simulink model "PowerCircuitPlant"  (R2020a)
settings: Solver=VariableStepAuto  StartTime=0.0  StopTime=10.0  RelTol=1e-3
libraries: fl_lib x5, nesl_utility x4, ee_lib x2
settings Model: DataDictionary=PCS_Simulation_EnviromentDD.sldd  Creator=ykamatan  LastModifiedBy=ykamatan

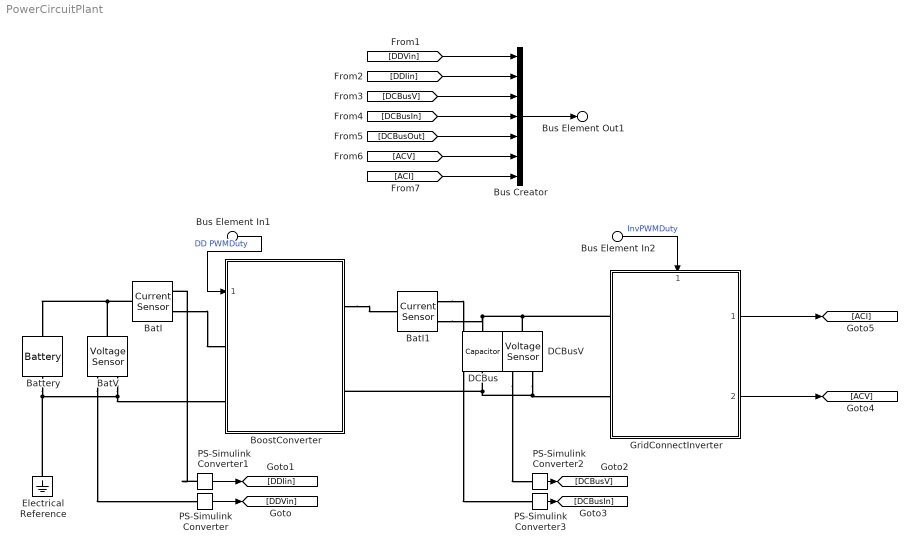
== system PowerCircuitPlant ==
  Bus Element In1 : Inport  PortName=DD PWMDuty
  Bus Element In2 : Inport  Port=2  PortName=InvPWMDuty
  BatI : fl_lib/Electrical/Electrical Sensors/Current Sensor
  BatI1 : fl_lib/Electrical/Electrical Sensors/Current Sensor
  BatV : fl_lib/Electrical/Electrical Sensors/Voltage Sensor
  Battery : ee_lib/Sources/Battery  Vnom=12 V  R1=2 Ohm  prm_AH=1  AH=50 hr*A  V1=11.5 V  AH1=25 hr*A  prm_R2=1  R2=2000 Ohm  prm_dyn=1  Rp1=0.005 Ohm  tau1=30 s  Rp2=0.005 Ohm  tau2=30 s  Rp3=0.005 Ohm  tau3=30 s  Rp4=0.005 Ohm  tau4=30 s  Rp5=0.005 Ohm  tau5=30 s  prm_fade=1  N_fade=100  AH_fade=45 hr*A  R1_fade=2.02 Ohm  V1_fade=10.35 V  i_specify=off  i_priority=None  i=0 A  i_nominal_specify=off  i_nominal_unit=A  i_nominal_value=1  v_specify=off  v_priority=None  v=0 V  v_nominal_specify=off  v_nominal_unit=V  v_nominal_value=1  charge_specify=off  charge_priority=High  charge=50 hr*A  charge_nominal_specify=off  charge_nominal_unit=hr*A  charge_nominal_value=1  num_cycles_specify=off  num_cycles_priority=High  num_cycles=0  num_cycles_nominal_specify=off  num_cycles_nominal_unit=1  num_cycles_nominal_value=1  thermal_mass=30000 J/K  Tmeas=298.15 K  Vnom_T2=12 V  R1_T2=2.2 Ohm  V1_T2=11.4 V  R2_T2=2200 Ohm  Rp1_T2=0.005 Ohm  tau1_T2=30 s  Rp2_T2=0.005 Ohm  tau2_T2=30 s  Rp3_T2=0.005 Ohm  tau3_T2=30 s  Rp4_T2=0.005 Ohm  tau4_T2=30 s  Rp5_T2=0.005 Ohm  tau5_T2=30 s  Tmeas2=273.15 K  temperature_specify=off  temperature_priority=High  temperature=298.15 K  temperature_nominal_specify=off  temperature_nominal_unit=K  temperature_nominal_value=1
  BoostConverter : Subsystem  ReferencedSubsystem=BoostConverter
  Bus Creator : BusCreator  Inputs=7
  DCBus : ee_lib/Passive/Capacitor  cap_option=0  c=1e-6 F  Cvec=[1e-05, 1e-06] F  Vvec=[0, 10] V  CV_table_symmetry=1  f_vec=[1, 10] kHz  DFext_vec=[.8, 1.2]  C_tol=5  enable_C_tol=0  tol_distribution=1  nSigma=4  r=1e-6 Ohm  g=0 1/Ohm  averaging_period=0 s  enable_operating_limits=0  operating_limit_action=2  max_working_voltage_range=[-25, 25] V  power_rating=1 W  enable_faults=0  fault_action=1  Cscale_faulted=100  R_faulted=1e-3 Ohm  G_faulted=0 1/Ohm  tau_fault=1e-3 s  enable_temporal_fault=0  t_fault=1 s  enable_behavioral_fault=0  max_permissible_voltage_range=[-100, 100] V  t_fail_on_voltage=1 s  i_specify=off  i_priority=None  i=0 A  i_nominal_specify=off  i_nominal_unit=A  i_nominal_value=1  v_specify=off  v_priority=None  v=0 V  v_nominal_specify=off  v_nominal_unit=V  v_nominal_value=1  vc_specify=off  vc_priority=High  vc=0 V  vc_nominal_specify=off  vc_nominal_unit=V  vc_nominal_value=1
  DCBusV : fl_lib/Electrical/Electrical Sensors/Voltage Sensor
  Electrical Reference : fl_lib/Electrical/Electrical Elements/Electrical Reference
  GridConnectInverter : Subsystem  ReferencedSubsystem=GridConnectInverter
      settings: PortSchema="{\"entries\":[{\"content\":{\"sides\":[{\"content\":{\"connectorIds\":[\"LConn1\",\"LConn2\"]},\"type\":\"ConnectorPlacement.EquallySpacedRectSide\",\"uuid\":\"5516e6e0-e90b-45b6-9097-7d81db5529b7\"},{\"content\":{\"connectorIds\":[\"Out1\",\"Out2\"],\"side\":\"RIGHT\"},\"type\":\"ConnectorPlacement.EquallySpacedRectSide\",\"uuid\":\"c08daa1d-3c8d-4022-a135-6251002e3faa\"},{\"content\":{\"connectorIds\":[\"In1\"],\"side\":\"TOP\"},\"type\":\"ConnectorPlacement.EquallySpacedRectSide\",\"uuid\":\"063f088e-77c7-44ca-915a-d9d0d7c33669\"}]},\"type\":\"ConnectorPlacement.EquallySpacedConnector\",\"uuid\":\"98f901b5-3d53-45dd-ae63-ab694af0ed2d\"}],\"packageUris\":[\"http://schema.mathworks.com/mf0/Connector/19700101\"],\"version\":\"1.0\"}"
  PS-Simulink Converter{,1..3} (4 alike) : nesl_utility/PS-Simulink Converter  PhysicalDomain=network_engine_domain  SubClassName=ps_output  LeftPortType=input  RightPortType=output  PseudoPeriodic=off  Frequencies=[]  Unit=inherit  AffineConversion=off
  Bus Element Out1 : Outport  PortName=SensorData
  wires:
  Bus Creator/1 -> Bus Element Out1/1
  [DDVin] -> Bus Creator/1
  [DDIin] -> Bus Creator/2
  [DCBusV] -> Bus Creator/3
  [DCBusIn] -> Bus Creator/4
  [DCBusOut] -> Bus Creator/5
  [ACV] -> Bus Creator/6
  [ACI] -> Bus Creator/7
  PS-Simulink Converter/1 -> [DDVin]
  PS-Simulink Converter1/1 -> [DDIin]
  PS-Simulink Converter2/1 -> [DCBusV]
  PS-Simulink Converter3/1 -> [DCBusIn]
  GridConnectInverter/2 -> [ACV]
  GridConnectInverter/1 -> [ACI]
  Bus Element In1/1 -> BoostConverter/1  "DD PWMDuty"
  Bus Element In2/1 -> GridConnectInverter/1  "InvPWMDuty"
  connections:
  DCBusV/LConn1 -- GridConnectInverter/LConn1 -- BatI1/RConn2 -- DCBus/LConn1
  BatV/LConn1 -- BatI/LConn1 -- Battery/LConn1
  BatV/RConn1 -- PS-Simulink Converter/LConn1
  PS-Simulink Converter1/LConn1 -- BatI/RConn1
  BatI1/RConn1 -- PS-Simulink Converter3/LConn1
  DCBusV/RConn1 -- PS-Simulink Converter2/LConn1
  BatI/RConn2 -- BoostConverter/LConn1
  BoostConverter/RConn1 -- BatI1/LConn1
  Electrical Reference/LConn1 -- Battery/RConn1 -- BatV/RConn2 -- BoostConverter/LConn2
  DCBusV/RConn2 -- GridConnectInverter/LConn2 -- BoostConverter/RConn2 -- DCBus/RConn1
